simulink model "Battery_Model_estimation"  (R2023a)
settings: Solver=VariableStepAuto  StartTime=0.0  StopTime=Sim_Time  RelTol=1e-3
undefined symbols (not defined in the file): Cn, I, ocv, R_Charge, R_Discharge, soc
settings Model: Creator=matha  LastModifiedBy=matha

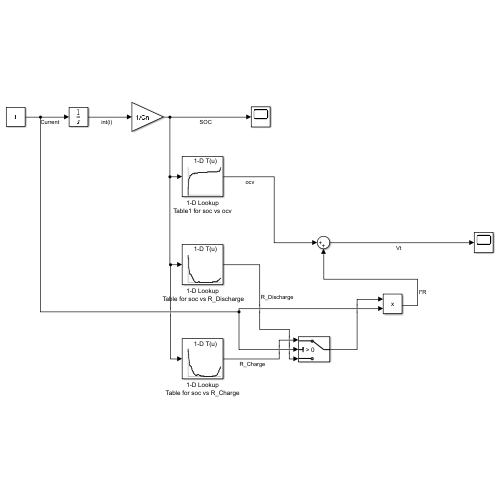
[thumbnail: Simulink's stored preview of the top-level diagram]
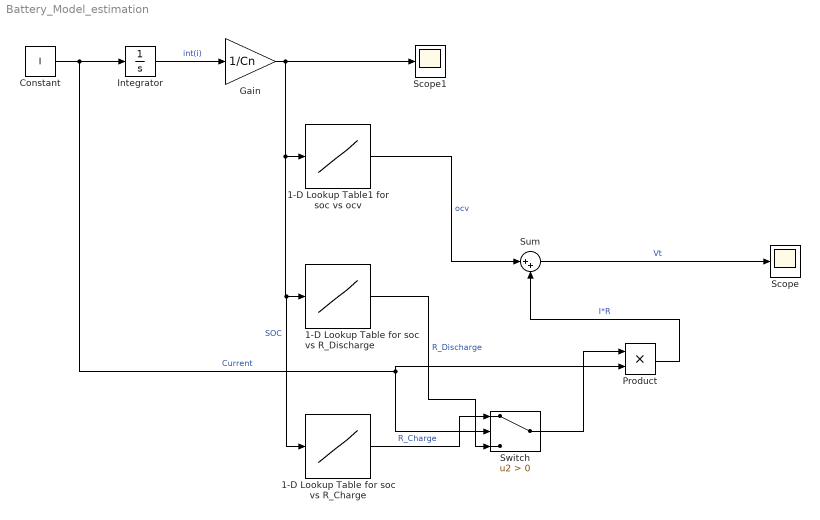
== system Battery_Model_estimation ==
  1-D Lookup Table for soc vs R_Discharge : Lookup_n-D  NumberOfTableDimensions=1  BreakpointsForDimension1=soc  Table=R_Discharge  InternalRulePriority=Speed  RndMeth=Simplest
  1-D Lookup Table for soc vs R_Charge : Lookup_n-D  NumberOfTableDimensions=1  BreakpointsForDimension1=soc  Table=R_Charge  InternalRulePriority=Speed  RndMeth=Simplest
  1-D Lookup Table1 for soc vs ocv : Lookup_n-D  NumberOfTableDimensions=1  BreakpointsForDimension1=soc  Table=ocv  InternalRulePriority=Speed  RndMeth=Simplest
  Constant : Constant  Value=I
  Gain : Gain  Gain=1/Cn
  Integrator : Integrator
  Product : Product
  Scope : Scope
  Scope1 : Scope
  Sum : Sum  Inputs=|++
  Switch : Switch  Criteria=u2 > Threshold  SaturateOnIntegerOverflow=off  InputSameDT=off
  wires:
  Constant/1 -> Switch/2, Product/2, Integrator/1  "Current"
  Integrator/1 -> Gain/1  "int(i)"
  Gain/1 -> Scope1/1, 1-D Lookup Table for soc vs R_Discharge/1, 1-D Lookup Table for soc vs R_Charge/1, 1-D Lookup Table1 for soc vs ocv/1  "SOC"
  1-D Lookup Table1 for soc vs ocv/1 -> Sum/1  "ocv"
  1-D Lookup Table for soc vs R_Discharge/1 -> Switch/3  "R_Discharge"
  Product/1 -> Sum/2  "I*R"
  Sum/1 -> Scope/1  "Vt"
  1-D Lookup Table for soc vs R_Charge/1 -> Switch/1  "R_Charge"
  Switch/1 -> Product/1
